simulink model "bic_3"  (R2018b)
settings: Solver=FixedStepAuto  StartTime=0.0  StopTime=1  FixedStep=Ts  RelTol=1e-5  EnableMultiTasking=on
values from neighbouring files (symbols this model uses):
  a_cmd = a    [sim_veh_MPC.m]
  delta_f = alpha    [sim_veh_MPC.m]
  psi0 = psi    (= 0)    [sim_veh_MPC.m]
  v_car0 = v    (= 1)    [sim_veh_MPC.m]
  x_car0 = x_car    (= -5)    [sim_veh_MPC.m]
  y_car0 = y_car    (= -5)    [sim_veh_MPC.m]
settings Model: Creator=Jesse  LastModifiedBy=Administrator
settings DataIOCC: LimitDataPoints=on
settings OptimizationCC: LifeSpan=inf
settings DebuggingCC: AllowSymbolicDim=off  LibraryContextMissingDiagnostic=none  SFUnexpectedBacktrackingDiag=warning  SFNoUnconditionalDefaultTransitionDiag=warning  SFExecutionAtInitializationDiag=none
settings ModelReferenceCC: PropagateSignalLabelsOutOfModel=off
settings SFSimCC: SimUseLocalCustomCode=off
settings RTWCC: RTWUseLocalCustomCode=off
settings CodeAppCC: StateflowObjectComments=on
settings GRTTargetCC: TargetLangStandard=C89/C90 (ANSI)
settings ConfigComp: CovMetricSettings=dw  CovHtmlReporting=on  CovSaveCumulativeToWorkspaceVar=on  CovSaveSingleToWorkspaceVar=on  CovExternalEMLEnable=off

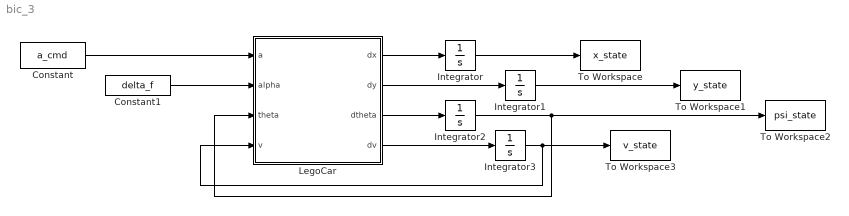
== system bic_3 ==
  Constant : Constant  Value=a_cmd
  Constant1 : Constant  Value=delta_f
  Integrator : Integrator  InitialCondition=x_car0
  Integrator1 : Integrator  InitialCondition=y_car0
  Integrator2 : Integrator  InitialCondition=psi0
  Integrator3 : Integrator  InitialCondition=v_car0
  LegoCar : MATLAB Function  TreatAsAtomicUnit=on
  To Workspace : ToWorkspace  VariableName=x_state  SaveFormat=Timeseries  SampleTime=-1
  To Workspace1 : ToWorkspace  VariableName=y_state  SaveFormat=Timeseries  SampleTime=-1
  To Workspace2 : ToWorkspace  VariableName=psi_state  SaveFormat=Timeseries  SampleTime=-1
  To Workspace3 : ToWorkspace  VariableName=v_state  SaveFormat=Timeseries  SampleTime=-1
  wires:
  LegoCar/3(dtheta) -> Integrator2/1
  Integrator2/1 -> LegoCar/3(theta), To Workspace2/1
  LegoCar/2(dy) -> Integrator1/1
  LegoCar/1(dx) -> Integrator/1
  Constant/1 -> LegoCar/1(a)
  Constant1/1 -> LegoCar/2(alpha)
  Integrator/1 -> To Workspace/1
  Integrator1/1 -> To Workspace1/1
  LegoCar/4(dv) -> Integrator3/1
  Integrator3/1 -> LegoCar/4(v), To Workspace3/1

== matlab function bic_3/LegoCar ==
  data: a input; dx output; alpha input; theta input; dy output; dtheta output; dv output; v input
function [dx,dy,dtheta,dv] = fcn(a,alpha,theta,v)
lr = 1.7;
lf = 1.5;
beta = atan(lr/(lr+lf)*tan(alpha));
dx = v*cos(theta+beta);
dy = v*sin(theta+beta);
dtheta = v/lr*tan(beta);
dv = a;
